simulink library "PRISMA"  (R2025b)
settings: Solver=VariableStepAuto  StartTime=0.0  StopTime=10.0  RelTol=1e-3
libraries: $bdroot x116, etargetslib x30, simulink x9
(part 2 of 3)

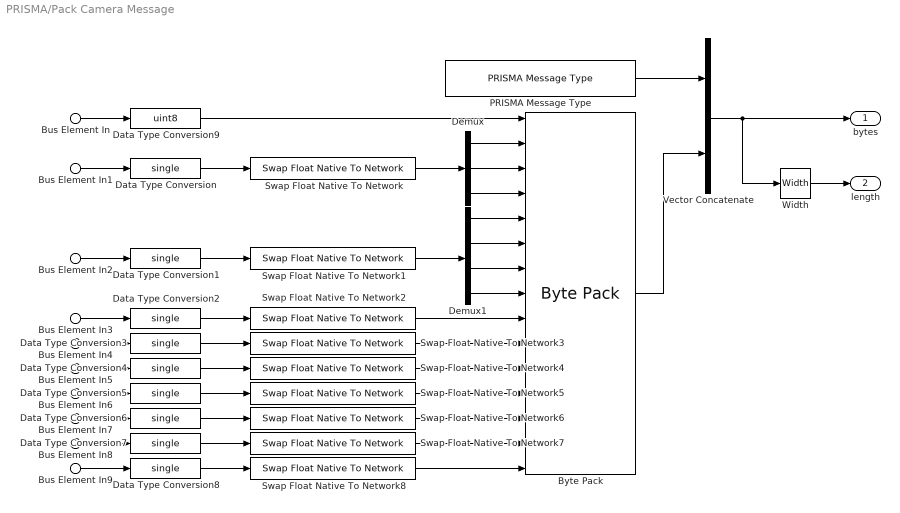
== system PRISMA/Pack Camera Message ==
  Bus Element In : Inport  PortName=camera  Element=mode
  Bus Element In1 : Inport  PortName=camera  Element=position
  Bus Element In2 : Inport  PortName=camera  Element=quaternion
  Bus Element In3 : Inport  PortName=camera  Element=clipNear
  Bus Element In4 : Inport  PortName=camera  Element=clipFar
  Bus Element In5 : Inport  PortName=camera  Element=orthographicLeft
  Bus Element In6 : Inport  PortName=camera  Element=orthographicRight
  Bus Element In7 : Inport  PortName=camera  Element=orthographicBottom
  Bus Element In8 : Inport  PortName=camera  Element=orthographicTop
  Bus Element In9 : Inport  PortName=camera  Element=perspectiveFieldOfView
  Byte Pack : etargetslib/Byte Pack  datatypes={'uint8','single','single','single','single','single','single','single','single','single','single','single','single','single','single'}  byteAlign=1
  Data Type Conversion{,1..8} (9 alike) : DataTypeConversion  OutDataTypeStr=single  SaturateOnIntegerOverflow=off  RndMeth=Floor
  Data Type Conversion9 : DataTypeConversion  OutDataTypeStr=uint8  SaturateOnIntegerOverflow=off  RndMeth=Floor
  Demux : Demux  Outputs=3
  Demux1 : Demux
  PRISMA Message Type : $bdroot/details/PRISMA Message Type  messageType=Camera
  Swap Float Native To Network{,1..8} (9 alike) : $bdroot/details/Swap Float Native To Network
  Vector Concatenate : Concatenate
  Width : Width  DataType=int32
  bytes : Outport  OutDataTypeStr=uint8
  length : Outport  Port=2  OutDataTypeStr=int32  PortDimensions=1
  wires:
  Bus Element In9/1 -> Data Type Conversion8/1
  Bus Element In8/1 -> Data Type Conversion7/1
  Bus Element In7/1 -> Data Type Conversion6/1
  Bus Element In6/1 -> Data Type Conversion5/1
  Bus Element In5/1 -> Data Type Conversion4/1
  Bus Element In4/1 -> Data Type Conversion3/1
  Bus Element In3/1 -> Data Type Conversion2/1
  Data Type Conversion6/1 -> Swap Float Native To Network6/1
  Data Type Conversion8/1 -> Swap Float Native To Network8/1
  Data Type Conversion7/1 -> Swap Float Native To Network7/1
  Data Type Conversion4/1 -> Swap Float Native To Network4/1
  Data Type Conversion5/1 -> Swap Float Native To Network5/1
  Data Type Conversion3/1 -> Swap Float Native To Network3/1
  Data Type Conversion2/1 -> Swap Float Native To Network2/1
  Bus Element In/1 -> Data Type Conversion9/1
  Bus Element In2/1 -> Data Type Conversion1/1
  Data Type Conversion1/1 -> Swap Float Native To Network1/1
  Demux1/4 -> Byte Pack/8
  Demux1/3 -> Byte Pack/7
  Demux1/2 -> Byte Pack/6
  Demux1/1 -> Byte Pack/5
  Bus Element In1/1 -> Data Type Conversion/1
  Demux/3 -> Byte Pack/4
  Demux/2 -> Byte Pack/3
  Demux/1 -> Byte Pack/2
  Data Type Conversion/1 -> Swap Float Native To Network/1
  PRISMA Message Type/1 -> Vector Concatenate/1
  Byte Pack/1 -> Vector Concatenate/2
  Vector Concatenate/1 -> Width/1, bytes/1
  Width/1 -> length/1
  Data Type Conversion9/1 -> Byte Pack/1
  Swap Float Native To Network/1 -> Demux/1
  Swap Float Native To Network1/1 -> Demux1/1
  Swap Float Native To Network2/1 -> Byte Pack/9
  Swap Float Native To Network3/1 -> Byte Pack/10
  Swap Float Native To Network4/1 -> Byte Pack/11
  Swap Float Native To Network5/1 -> Byte Pack/12
  Swap Float Native To Network6/1 -> Byte Pack/13
  Swap Float Native To Network7/1 -> Byte Pack/14
  Swap Float Native To Network8/1 -> Byte Pack/15

== system PRISMA/Pack Clear Message ==
  PRISMA Message Type : $bdroot/details/PRISMA Message Type  messageType=Clear
  Width : Width  DataType=int32
  bytes : Outport  OutDataTypeStr=uint8
  length : Outport  Port=2  OutDataTypeStr=int32  PortDimensions=1
  wires:
  Width/1 -> length/1
  PRISMA Message Type/1 -> bytes/1, Width/1

== system PRISMA/Pack Directional Light Message ==
  Bus Element In : Inport  PortName=directionalLight  Element=shouldBeDeleted
  Bus Element In1 : Inport  PortName=directionalLight  Element=directionalLightID
  Bus Element In2 : Inport  PortName=directionalLight  Element=visible
  Bus Element In3 : Inport  PortName=directionalLight  Element=color
  Bus Element In4 : Inport  PortName=directionalLight  Element=direction
  Byte Pack : etargetslib/Byte Pack  datatypes={'uint32','uint8','single','single','single','single','single','single'}  byteAlign=1
  Constant : Constant  Value=false  OutDataTypeStr=boolean
  Data Type Conversion : DataTypeConversion  OutDataTypeStr=single  SaturateOnIntegerOverflow=off  RndMeth=Floor
  Data Type Conversion1 : DataTypeConversion  OutDataTypeStr=uint32  SaturateOnIntegerOverflow=off  RndMeth=Floor
  Data Type Conversion2 : DataTypeConversion  OutDataTypeStr=single  SaturateOnIntegerOverflow=off  RndMeth=Floor
  Data Type Conversion3 : DataTypeConversion  OutDataTypeStr=boolean  SaturateOnIntegerOverflow=off  RndMeth=Floor
  Data Type Conversion4 : DataTypeConversion  OutDataTypeStr=boolean  SaturateOnIntegerOverflow=off  RndMeth=Floor
  Demux : Demux  Outputs=3
  Demux1 : Demux  Outputs=3
  Mux : Mux  Inputs=8
  PRISMA Bitfield To Byte : $bdroot/details/PRISMA Bitfield To Byte
  PRISMA Message Type : $bdroot/details/PRISMA Message Type  messageType=Directional Light
  Swap Float Native To Network : $bdroot/details/Swap Float Native To Network
  Swap Float Native To Network1 : $bdroot/details/Swap Float Native To Network
  Swap Uint32 Native To Network : $bdroot/details/Swap Uint32 Native To Network
  Vector Concatenate : Concatenate
  Width : Width  DataType=int32
  bytes : Outport  OutDataTypeStr=uint8
  length : Outport  Port=2  OutDataTypeStr=int32  PortDimensions=1
  wires:
  Bus Element In4/1 -> Data Type Conversion2/1
  Bus Element In3/1 -> Data Type Conversion/1
  Demux1/1 -> Byte Pack/6
  Demux1/2 -> Byte Pack/7
  Demux1/3 -> Byte Pack/8
  Demux/1 -> Byte Pack/3
  Demux/2 -> Byte Pack/4
  Demux/3 -> Byte Pack/5
  Data Type Conversion2/1 -> Swap Float Native To Network1/1
  Bus Element In2/1 -> Data Type Conversion4/1
  Bus Element In/1 -> Data Type Conversion3/1
  PRISMA Bitfield To Byte/1 -> Byte Pack/2
  Constant/1 -> Mux/8, Mux/3, Mux/4, Mux/5, Mux/6, Mux/7
  Mux/1 -> PRISMA Bitfield To Byte/1
  Bus Element In1/1 -> Data Type Conversion1/1
  Data Type Conversion1/1 -> Swap Uint32 Native To Network/1
  Data Type Conversion/1 -> Swap Float Native To Network/1
  PRISMA Message Type/1 -> Vector Concatenate/1
  Byte Pack/1 -> Vector Concatenate/2
  Vector Concatenate/1 -> Width/1, bytes/1
  Width/1 -> length/1
  Data Type Conversion3/1 -> Mux/1
  Data Type Conversion4/1 -> Mux/2
  Swap Uint32 Native To Network/1 -> Byte Pack/1
  Swap Float Native To Network/1 -> Demux/1
  Swap Float Native To Network1/1 -> Demux1/1

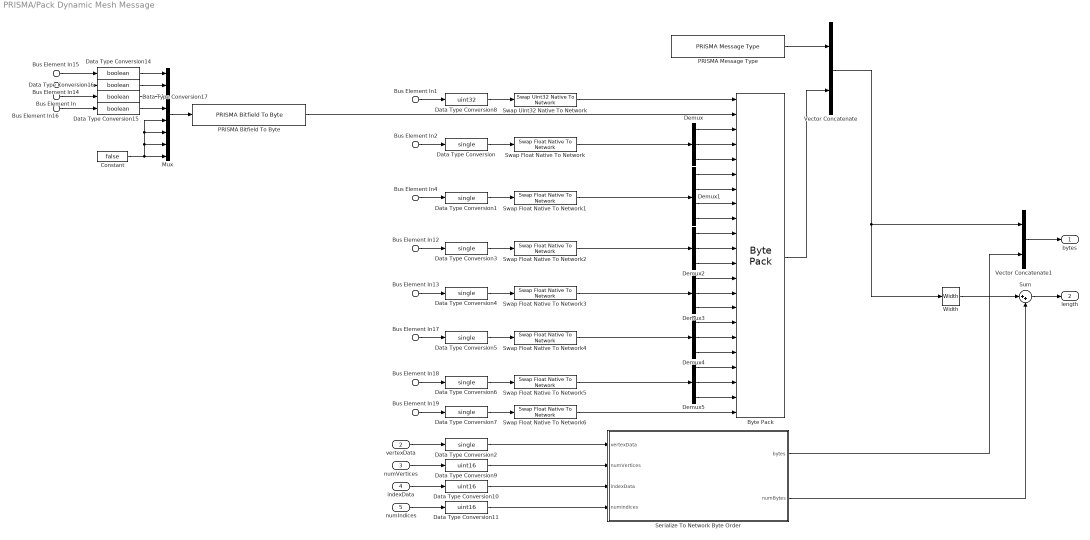
== system PRISMA/Pack Dynamic Mesh Message ==
  Bus Element In14 : Inport  PortName=dynamicMesh  Element=updateMesh
  Bus Element In : Inport  PortName=dynamicMesh  Element=visible
  Bus Element In15 : Inport  PortName=dynamicMesh  Element=shouldBeDeleted
  Bus Element In16 : Inport  PortName=dynamicMesh  Element=castShadow
  Bus Element In1 : Inport  PortName=dynamicMesh  Element=meshID
  Bus Element In2 : Inport  PortName=dynamicMesh  Element=position
  Bus Element In4 : Inport  PortName=dynamicMesh  Element=quaternion
  Bus Element In12 : Inport  PortName=dynamicMesh  Element=scale
  Bus Element In13 : Inport  PortName=dynamicMesh  Element=diffuseColorMultiplier
  Bus Element In17 : Inport  PortName=dynamicMesh  Element=specularColorMultiplier
  Bus Element In18 : Inport  PortName=dynamicMesh  Element=emissionColorMultiplier
  Bus Element In19 : Inport  PortName=dynamicMesh  Element=shininessMultiplier
  vertexData : Inport  Port=2  PortDimensions=[6,2000]
  numVertices : Inport  Port=3  PortDimensions=1
  indexData : Inport  Port=4  PortDimensions=10000
  numIndices : Inport  Port=5  PortDimensions=1
  Byte Pack : etargetslib/Byte Pack  datatypes={'uint32','uint8','single','single','single','single','single','single','single','single','single','single','single','single','single','single','single','single','single','single','single','single'}  byteAlign=1
  Constant : Constant  Value=false  OutDataTypeStr=boolean
  Data Type Conversion{,1..7} (8 alike) : DataTypeConversion  OutDataTypeStr=single  SaturateOnIntegerOverflow=off  RndMeth=Floor
  Data Type Conversion10 : DataTypeConversion  OutDataTypeStr=uint16  SaturateOnIntegerOverflow=off  RndMeth=Floor
  Data Type Conversion11 : DataTypeConversion  OutDataTypeStr=uint16  SaturateOnIntegerOverflow=off  RndMeth=Floor
  Data Type Conversion{14..17} (4 alike) : DataTypeConversion  OutDataTypeStr=boolean  SaturateOnIntegerOverflow=off  RndMeth=Floor
  Data Type Conversion8 : DataTypeConversion  OutDataTypeStr=uint32  SaturateOnIntegerOverflow=off  RndMeth=Floor
  Data Type Conversion9 : DataTypeConversion  OutDataTypeStr=uint16  SaturateOnIntegerOverflow=off  RndMeth=Floor
  Demux{,2..5} (5 alike) : Demux  Outputs=3
  Demux1 : Demux
  Mux : Mux  Inputs=8
  PRISMA Bitfield To Byte : $bdroot/details/PRISMA Bitfield To Byte
  PRISMA Message Type : $bdroot/details/PRISMA Message Type  messageType=Dynamic Mesh
  Serialize To Network Byte Order : MATLAB Function  TreatAsAtomicUnit=on
  Sum : Sum  Inputs=|++
  Swap Float Native To Network{,1..6} (7 alike) : $bdroot/details/Swap Float Native To Network
  Swap Uint32 Native To Network : $bdroot/details/Swap Uint32 Native To Network
  Vector Concatenate : Concatenate
  Vector Concatenate1 : Concatenate
  Width : Width  DataType=int32
  bytes : Outport  OutDataTypeStr=uint8
  length : Outport  Port=2  OutDataTypeStr=int32  PortDimensions=1
  wires:
  Bus Element In14/1 -> Data Type Conversion16/1
  Constant/1 -> Mux/7, Mux/6, Mux/5, Mux/8
  Mux/1 -> PRISMA Bitfield To Byte/1
  Vector Concatenate/1 -> Vector Concatenate1/1, Width/1
  Vector Concatenate1/1 -> bytes/1
  Serialize To Network Byte Order/2(numBytes) -> Sum/2
  Serialize To Network Byte Order/1(bytes) -> Vector Concatenate1/2
  Byte Pack/1 -> Vector Concatenate/2
  Sum/1 -> length/1
  Width/1 -> Sum/1
  Bus Element In/1 -> Data Type Conversion17/1
  PRISMA Message Type/1 -> Vector Concatenate/1
  Data Type Conversion16/1 -> Mux/2
  Data Type Conversion17/1 -> Mux/3
  Data Type Conversion14/1 -> Mux/1
  Bus Element In15/1 -> Data Type Conversion14/1
  Bus Element In16/1 -> Data Type Conversion15/1
  Data Type Conversion15/1 -> Mux/4
  Bus Element In13/1 -> Data Type Conversion4/1
  Bus Element In17/1 -> Data Type Conversion5/1
  Bus Element In19/1 -> Data Type Conversion7/1
  Data Type Conversion7/1 -> Swap Float Native To Network6/1
  Demux1/4 -> Byte Pack/9
  Demux1/1 -> Byte Pack/6
  Demux3/3 -> Byte Pack/15
  Demux1/3 -> Byte Pack/8
  Demux/2 -> Byte Pack/4
  Demux/3 -> Byte Pack/5
  Demux/1 -> Byte Pack/3
  Data Type Conversion6/1 -> Swap Float Native To Network5/1
  Demux3/2 -> Byte Pack/14
  Demux2/3 -> Byte Pack/12
  Demux2/2 -> Byte Pack/11
  Data Type Conversion8/1 -> Swap Uint32 Native To Network/1
  Demux4/2 -> Byte Pack/17
  Data Type Conversion5/1 -> Swap Float Native To Network4/1
  Bus Element In2/1 -> Data Type Conversion/1
  Data Type Conversion3/1 -> Swap Float Native To Network2/1
  Demux5/3 -> Byte Pack/21
  Demux5/2 -> Byte Pack/20
  Bus Element In1/1 -> Data Type Conversion8/1
  Demux2/1 -> Byte Pack/10
  Demux3/1 -> Byte Pack/13
  Demux5/1 -> Byte Pack/19
  PRISMA Bitfield To Byte/1 -> Byte Pack/2
  Data Type Conversion/1 -> Swap Float Native To Network/1
  Demux1/2 -> Byte Pack/7
  Bus Element In18/1 -> Data Type Conversion6/1
  Data Type Conversion4/1 -> Swap Float Native To Network3/1
  Demux4/3 -> Byte Pack/18
  Data Type Conversion1/1 -> Swap Float Native To Network1/1
  Bus Element In4/1 -> Data Type Conversion1/1
  Demux4/1 -> Byte Pack/16
  Bus Element In12/1 -> Data Type Conversion3/1
  vertexData/1 -> Data Type Conversion2/1
  numVertices/1 -> Data Type Conversion9/1
  indexData/1 -> Data Type Conversion10/1
  numIndices/1 -> Data Type Conversion11/1
  Swap Uint32 Native To Network/1 -> Byte Pack/1
  Swap Float Native To Network/1 -> Demux/1
  Swap Float Native To Network1/1 -> Demux1/1
  Swap Float Native To Network2/1 -> Demux2/1
  Swap Float Native To Network3/1 -> Demux3/1
  Swap Float Native To Network4/1 -> Demux4/1
  Swap Float Native To Network5/1 -> Demux5/1
  Swap Float Native To Network6/1 -> Byte Pack/22
  Data Type Conversion2/1 -> Serialize To Network Byte Order/1(vertexData)
  Data Type Conversion9/1 -> Serialize To Network Byte Order/2(numVertices)
  Data Type Conversion10/1 -> Serialize To Network Byte Order/3(indexData)
  Data Type Conversion11/1 -> Serialize To Network Byte Order/4(numIndices)

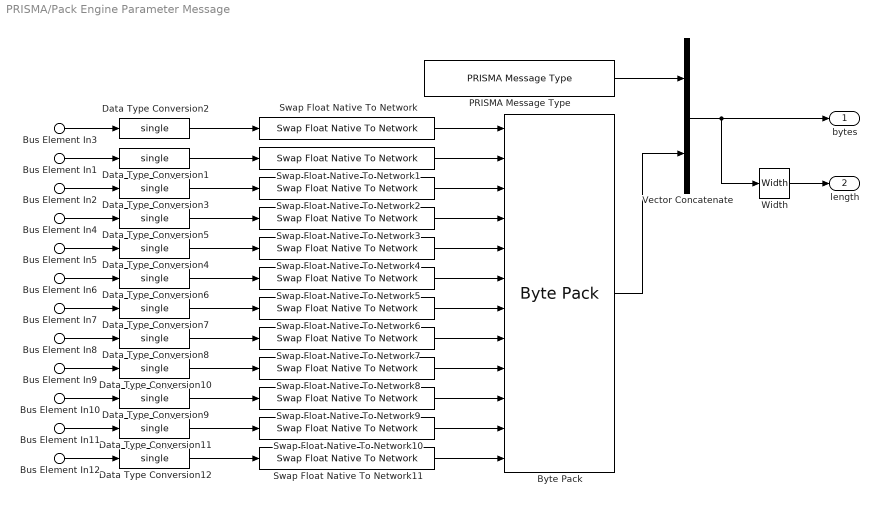
== system PRISMA/Pack Engine Parameter Message ==
  Bus Element In3 : Inport  PortName=engineParameter  Element=ambientOcclusionRadius
  Bus Element In1 : Inport  PortName=engineParameter  Element=ambientOcclusionBias
  Bus Element In2 : Inport  PortName=engineParameter  Element=ambientOcclusionEnhance
  Bus Element In4 : Inport  PortName=engineParameter  Element=removeShadowOnWater
  Bus Element In5 : Inport  PortName=engineParameter  Element=bloomBrightnessThreshold
  Bus Element In6 : Inport  PortName=engineParameter  Element=bloomStrength
  Bus Element In7 : Inport  PortName=engineParameter  Element=gamma
  Bus Element In8 : Inport  PortName=engineParameter  Element=ditheringNoiseGranularity
  Bus Element In9 : Inport  PortName=engineParameter  Element=shadowBiasMin
  Bus Element In10 : Inport  PortName=engineParameter  Element=shadowBiasMax
  Bus Element In11 : Inport  PortName=engineParameter  Element=exposure
  Bus Element In12 : Inport  PortName=engineParameter  Element=toneMappingStrength
  Byte Pack : etargetslib/Byte Pack  datatypes={'single','single','single','single','single','single','single','single','single','single','single','single'}  byteAlign=1
  Data Type Conversion{1..12} (12 alike) : DataTypeConversion  OutDataTypeStr=single  SaturateOnIntegerOverflow=off  RndMeth=Floor
  PRISMA Message Type : $bdroot/details/PRISMA Message Type  messageType=Engine Parameter
  Swap Float Native To Network{,1..11} (12 alike) : $bdroot/details/Swap Float Native To Network
  Vector Concatenate : Concatenate
  Width : Width  DataType=int32
  bytes : Outport  OutDataTypeStr=uint8
  length : Outport  Port=2  OutDataTypeStr=int32  PortDimensions=1
  wires:
  Bus Element In12/1 -> Data Type Conversion12/1
  Bus Element In11/1 -> Data Type Conversion11/1
  Bus Element In10/1 -> Data Type Conversion9/1
  Bus Element In9/1 -> Data Type Conversion10/1
  Bus Element In8/1 -> Data Type Conversion8/1
  Bus Element In7/1 -> Data Type Conversion7/1
  Bus Element In6/1 -> Data Type Conversion6/1
  Bus Element In5/1 -> Data Type Conversion4/1
  Bus Element In4/1 -> Data Type Conversion5/1
  Bus Element In2/1 -> Data Type Conversion3/1
  Bus Element In1/1 -> Data Type Conversion1/1
  Width/1 -> length/1
  Vector Concatenate/1 -> bytes/1, Width/1
  Byte Pack/1 -> Vector Concatenate/2
  PRISMA Message Type/1 -> Vector Concatenate/1
  Bus Element In3/1 -> Data Type Conversion2/1
  Data Type Conversion2/1 -> Swap Float Native To Network/1
  Data Type Conversion1/1 -> Swap Float Native To Network1/1
  Data Type Conversion3/1 -> Swap Float Native To Network2/1
  Data Type Conversion5/1 -> Swap Float Native To Network3/1
  Data Type Conversion4/1 -> Swap Float Native To Network4/1
  Data Type Conversion6/1 -> Swap Float Native To Network5/1
  Data Type Conversion7/1 -> Swap Float Native To Network6/1
  Data Type Conversion8/1 -> Swap Float Native To Network7/1
  Data Type Conversion10/1 -> Swap Float Native To Network8/1
  Data Type Conversion9/1 -> Swap Float Native To Network9/1
  Data Type Conversion11/1 -> Swap Float Native To Network10/1
  Data Type Conversion12/1 -> Swap Float Native To Network11/1
  Swap Float Native To Network/1 -> Byte Pack/1
  Swap Float Native To Network1/1 -> Byte Pack/2
  Swap Float Native To Network2/1 -> Byte Pack/3
  Swap Float Native To Network3/1 -> Byte Pack/4
  Swap Float Native To Network4/1 -> Byte Pack/5
  Swap Float Native To Network5/1 -> Byte Pack/6
  Swap Float Native To Network6/1 -> Byte Pack/7
  Swap Float Native To Network7/1 -> Byte Pack/8
  Swap Float Native To Network8/1 -> Byte Pack/9
  Swap Float Native To Network9/1 -> Byte Pack/10
  Swap Float Native To Network10/1 -> Byte Pack/11
  Swap Float Native To Network11/1 -> Byte Pack/12

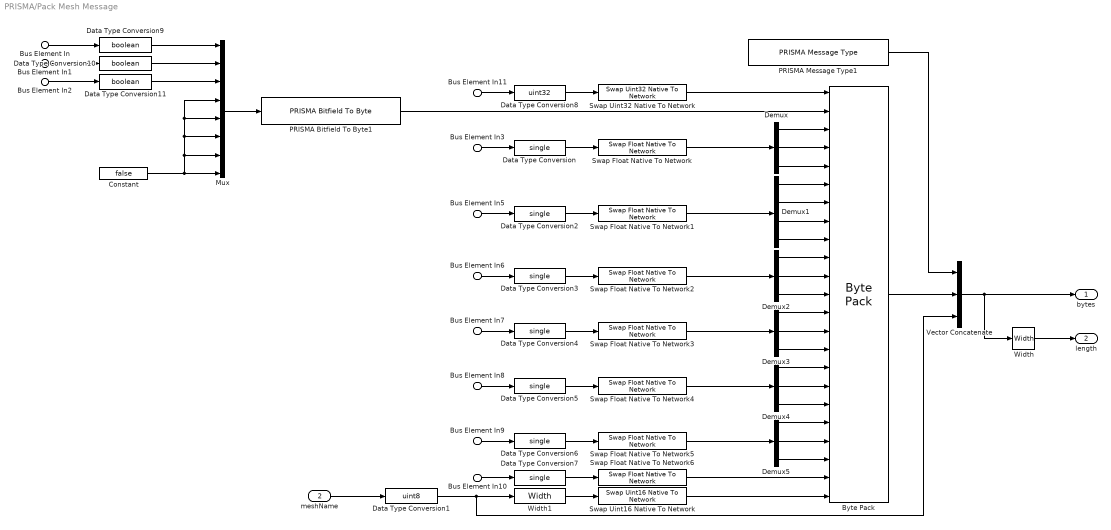
== system PRISMA/Pack Mesh Message ==
  Bus Element In : Inport  PortName=mesh  Element=shouldBeDeleted
  Bus Element In1 : Inport  PortName=mesh  Element=visible
  Bus Element In2 : Inport  PortName=mesh  Element=castShadow
  Bus Element In3 : Inport  PortName=mesh  Element=position
  Bus Element In5 : Inport  PortName=mesh  Element=quaternion
  Bus Element In6 : Inport  PortName=mesh  Element=scale
  Bus Element In7 : Inport  PortName=mesh  Element=diffuseColorMultiplier
  Bus Element In8 : Inport  PortName=mesh  Element=specularColorMultiplier
  Bus Element In9 : Inport  PortName=mesh  Element=emissionColorMultiplier
  Bus Element In10 : Inport  PortName=mesh  Element=shininessMultiplier
  Bus Element In11 : Inport  PortName=mesh  Element=meshID
  meshName : Inport  Port=2  OutDataTypeStr=uint8
  Byte Pack : etargetslib/Byte Pack  datatypes={'uint32','uint8','single','single','single','single','single','single','single','single','single','single','single','single','single','single','single','single','single','single','single','single','uint16'}  byteAlign=1
  Constant : Constant  Value=false  OutDataTypeStr=boolean
  Data Type Conversion{,2..7} (7 alike) : DataTypeConversion  OutDataTypeStr=single  SaturateOnIntegerOverflow=off  RndMeth=Floor
  Data Type Conversion1 : DataTypeConversion  OutDataTypeStr=uint8  SaturateOnIntegerOverflow=off  RndMeth=Floor
  Data Type Conversion10 : DataTypeConversion  OutDataTypeStr=boolean  SaturateOnIntegerOverflow=off  RndMeth=Floor
  Data Type Conversion11 : DataTypeConversion  OutDataTypeStr=boolean  SaturateOnIntegerOverflow=off  RndMeth=Floor
  Data Type Conversion8 : DataTypeConversion  OutDataTypeStr=uint32  SaturateOnIntegerOverflow=off  RndMeth=Floor
  Data Type Conversion9 : DataTypeConversion  OutDataTypeStr=boolean  SaturateOnIntegerOverflow=off  RndMeth=Floor
  Demux{,2..5} (5 alike) : Demux  Outputs=3
  Demux1 : Demux
  Mux : Mux  Inputs=8
  PRISMA Bitfield To Byte1 : $bdroot/details/PRISMA Bitfield To Byte
  PRISMA Message Type1 : $bdroot/details/PRISMA Message Type  messageType=Mesh
  Swap Float Native To Network{,1..6} (7 alike) : $bdroot/details/Swap Float Native To Network
  Swap Uint16 Native To Network : $bdroot/details/Swap Uint16 Native To Network
  Swap Uint32 Native To Network : $bdroot/details/Swap Uint32 Native To Network
  Vector Concatenate : Concatenate  NumInputs=3
  Width : Width  DataType=int32
  Width1 : Width  DataType=uint16
  bytes : Outport  OutDataTypeStr=uint8
  length : Outport  Port=2  OutDataTypeStr=int32  PortDimensions=1
  wires:
  Data Type Conversion8/1 -> Swap Uint32 Native To Network/1
  Bus Element In10/1 -> Data Type Conversion7/1
  Bus Element In9/1 -> Data Type Conversion6/1
  Bus Element In8/1 -> Data Type Conversion5/1
  Bus Element In7/1 -> Data Type Conversion4/1
  Bus Element In6/1 -> Data Type Conversion3/1
  Bus Element In5/1 -> Data Type Conversion2/1
  Bus Element In3/1 -> Data Type Conversion/1
  Bus Element In2/1 -> Data Type Conversion11/1
  Bus Element In/1 -> Data Type Conversion9/1
  Width/1 -> length/1
  Vector Concatenate/1 -> bytes/1, Width/1
  Width1/1 -> Swap Uint16 Native To Network/1
  Data Type Conversion7/1 -> Swap Float Native To Network6/1
  Data Type Conversion6/1 -> Swap Float Native To Network5/1
  Data Type Conversion5/1 -> Swap Float Native To Network4/1
  Data Type Conversion4/1 -> Swap Float Native To Network3/1
  Data Type Conversion3/1 -> Swap Float Native To Network2/1
  Data Type Conversion2/1 -> Swap Float Native To Network1/1
  Data Type Conversion/1 -> Swap Float Native To Network/1
  Mux/1 -> PRISMA Bitfield To Byte1/1
  Constant/1 -> Mux/4, Mux/5, Mux/6, Mux/7, Mux/8
  Bus Element In1/1 -> Data Type Conversion10/1
  PRISMA Bitfield To Byte1/1 -> Byte Pack/2
  meshName/1 -> Data Type Conversion1/1
  Demux5/3 -> Byte Pack/21
  Demux5/2 -> Byte Pack/20
  Demux5/1 -> Byte Pack/19
  Demux4/1 -> Byte Pack/16
  Demux4/2 -> Byte Pack/17
  Demux4/3 -> Byte Pack/18
  Demux3/3 -> Byte Pack/15
  Demux3/2 -> Byte Pack/14
  Demux3/1 -> Byte Pack/13
  Demux2/1 -> Byte Pack/10
  Demux2/2 -> Byte Pack/11
  Demux2/3 -> Byte Pack/12
  Demux/3 -> Byte Pack/5
  Demux/2 -> Byte Pack/4
  Demux/1 -> Byte Pack/3
  Byte Pack/1 -> Vector Concatenate/2
  PRISMA Message Type1/1 -> Vector Concatenate/1
  Bus Element In11/1 -> Data Type Conversion8/1
  Demux1/4 -> Byte Pack/9
  Demux1/3 -> Byte Pack/8
  Demux1/2 -> Byte Pack/7
  Demux1/1 -> Byte Pack/6
  Data Type Conversion1/1 -> Vector Concatenate/3, Width1/1
  Data Type Conversion9/1 -> Mux/1
  Data Type Conversion10/1 -> Mux/2
  Data Type Conversion11/1 -> Mux/3
  Swap Uint32 Native To Network/1 -> Byte Pack/1
  Swap Float Native To Network/1 -> Demux/1
  Swap Float Native To Network1/1 -> Demux1/1
  Swap Float Native To Network2/1 -> Demux2/1
  Swap Float Native To Network3/1 -> Demux3/1
  Swap Float Native To Network4/1 -> Demux4/1
  Swap Float Native To Network5/1 -> Demux5/1
  Swap Float Native To Network6/1 -> Byte Pack/22
  Swap Uint16 Native To Network/1 -> Byte Pack/23

== system PRISMA/Pack Point Light Message ==
  Bus Element In : Inport  PortName=pointLight  Element=shouldBeDeleted
  Bus Element In1 : Inport  PortName=pointLight  Element=pointLightID
  Bus Element In2 : Inport  PortName=pointLight  Element=visible
  Bus Element In3 : Inport  PortName=pointLight  Element=color
  Bus Element In4 : Inport  PortName=pointLight  Element=position
  Bus Element In5 : Inport  PortName=pointLight  Element=quadraticFalloff
  Bus Element In6 : Inport  PortName=pointLight  Element=invRadiusPow4
  Byte Pack : etargetslib/Byte Pack  datatypes={'uint32','uint8','single','single','single','single','single','single','single','single'}  byteAlign=1
  Constant : Constant  Value=false  OutDataTypeStr=boolean
  Data Type Conversion{,2..4} (4 alike) : DataTypeConversion  OutDataTypeStr=single  SaturateOnIntegerOverflow=off  RndMeth=Floor
  Data Type Conversion1 : DataTypeConversion  OutDataTypeStr=uint32  SaturateOnIntegerOverflow=off  RndMeth=Floor
  Data Type Conversion5 : DataTypeConversion  OutDataTypeStr=boolean  SaturateOnIntegerOverflow=off  RndMeth=Floor
  Data Type Conversion6 : DataTypeConversion  OutDataTypeStr=boolean  SaturateOnIntegerOverflow=off  RndMeth=Floor
  Demux1 : Demux  Outputs=3
  Demux2 : Demux  Outputs=3
  Mux : Mux  Inputs=8
  PRISMA Bitfield To Byte : $bdroot/details/PRISMA Bitfield To Byte
  PRISMA Message Type : $bdroot/details/PRISMA Message Type  messageType=Point Light
  Swap Float Native To Network{,1..3} (4 alike) : $bdroot/details/Swap Float Native To Network
  Swap Uint32 Native To Network : $bdroot/details/Swap Uint32 Native To Network
  Vector Concatenate : Concatenate
  Width : Width  DataType=int32
  bytes : Outport  OutDataTypeStr=uint8
  length : Outport  Port=2  OutDataTypeStr=int32  PortDimensions=1
  wires:
  Data Type Conversion/1 -> Swap Float Native To Network/1
  Demux2/3 -> Byte Pack/5
  Demux2/2 -> Byte Pack/4
  Demux2/1 -> Byte Pack/3
  Data Type Conversion4/1 -> Swap Float Native To Network3/1
  Bus Element In6/1 -> Data Type Conversion4/1
  Bus Element In5/1 -> Data Type Conversion3/1
  Data Type Conversion3/1 -> Swap Float Native To Network2/1
  Width/1 -> length/1
  Vector Concatenate/1 -> bytes/1, Width/1
  Byte Pack/1 -> Vector Concatenate/2
  PRISMA Message Type/1 -> Vector Concatenate/1
  Data Type Conversion1/1 -> Swap Uint32 Native To Network/1
  Bus Element In1/1 -> Data Type Conversion1/1
  Mux/1 -> PRISMA Bitfield To Byte/1
  Constant/1 -> Mux/7, Mux/6, Mux/5, Mux/4, Mux/3, Mux/8
  PRISMA Bitfield To Byte/1 -> Byte Pack/2
  Bus Element In/1 -> Data Type Conversion5/1
  Bus Element In2/1 -> Data Type Conversion6/1
  Data Type Conversion2/1 -> Swap Float Native To Network1/1
  Demux1/3 -> Byte Pack/8
  Demux1/2 -> Byte Pack/7
  Demux1/1 -> Byte Pack/6
  Bus Element In3/1 -> Data Type Conversion/1
  Bus Element In4/1 -> Data Type Conversion2/1
  Data Type Conversion5/1 -> Mux/1
  Data Type Conversion6/1 -> Mux/2
  Swap Uint32 Native To Network/1 -> Byte Pack/1
  Swap Float Native To Network/1 -> Demux2/1
  Swap Float Native To Network1/1 -> Demux1/1
  Swap Float Native To Network2/1 -> Byte Pack/9
  Swap Float Native To Network3/1 -> Byte Pack/10

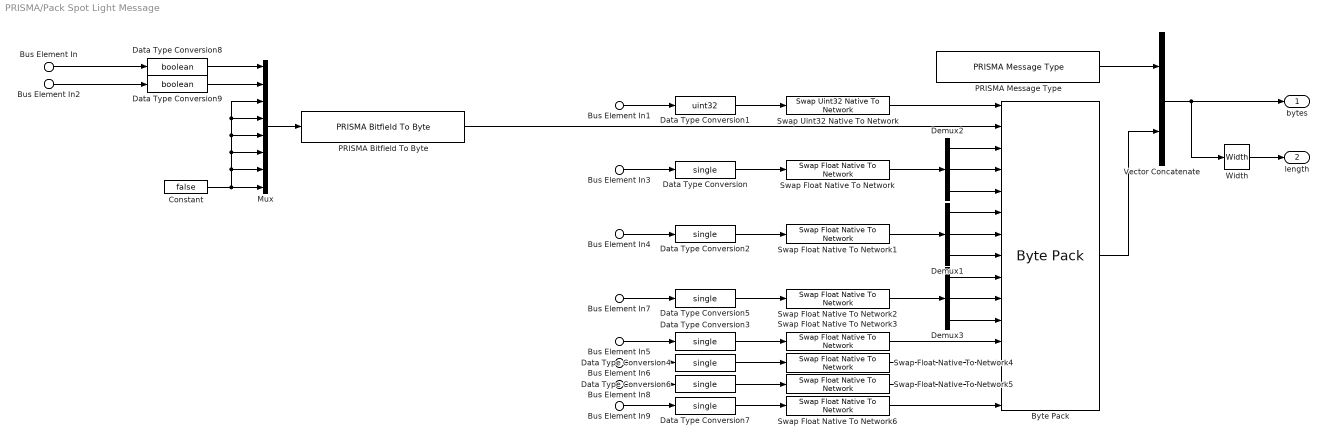
== system PRISMA/Pack Spot Light Message ==
  Bus Element In : Inport  PortName=spotLight  Element=shouldBeDeleted
  Bus Element In1 : Inport  PortName=spotLight  Element=spotLightID
  Bus Element In2 : Inport  PortName=spotLight  Element=visible
  Bus Element In3 : Inport  PortName=spotLight  Element=color
  Bus Element In4 : Inport  PortName=spotLight  Element=position
  Bus Element In5 : Inport  PortName=spotLight  Element=quadraticFalloff
  Bus Element In6 : Inport  PortName=spotLight  Element=invRadiusPow4
  Bus Element In7 : Inport  PortName=spotLight  Element=direction
  Bus Element In8 : Inport  PortName=spotLight  Element=cosInnerCutOffAngle
  Bus Element In9 : Inport  PortName=spotLight  Element=cosOuterCutOffAngle
  Byte Pack : etargetslib/Byte Pack  datatypes={'uint32','uint8','single','single','single','single','single','single','single','single','single','single','single','single','single'}  byteAlign=1
  Constant : Constant  Value=false  OutDataTypeStr=boolean
  Data Type Conversion{,2..7} (7 alike) : DataTypeConversion  OutDataTypeStr=single  SaturateOnIntegerOverflow=off  RndMeth=Floor
  Data Type Conversion1 : DataTypeConversion  OutDataTypeStr=uint32  SaturateOnIntegerOverflow=off  RndMeth=Floor
  Data Type Conversion8 : DataTypeConversion  OutDataTypeStr=boolean  SaturateOnIntegerOverflow=off  RndMeth=Floor
  Data Type Conversion9 : DataTypeConversion  OutDataTypeStr=boolean  SaturateOnIntegerOverflow=off  RndMeth=Floor
  Demux1 : Demux  Outputs=3
  Demux2 : Demux  Outputs=3
  Demux3 : Demux  Outputs=3
  Mux : Mux  Inputs=8
  PRISMA Bitfield To Byte : $bdroot/details/PRISMA Bitfield To Byte
  PRISMA Message Type : $bdroot/details/PRISMA Message Type  messageType=Spot Light
  Swap Float Native To Network{,1..6} (7 alike) : $bdroot/details/Swap Float Native To Network
  Swap Uint32 Native To Network : $bdroot/details/Swap Uint32 Native To Network
  Vector Concatenate : Concatenate
  Width : Width  DataType=int32
  bytes : Outport  OutDataTypeStr=uint8
  length : Outport  Port=2  OutDataTypeStr=int32  PortDimensions=1
  wires:
  Bus Element In9/1 -> Data Type Conversion7/1
  Bus Element In8/1 -> Data Type Conversion6/1
  Data Type Conversion6/1 -> Swap Float Native To Network5/1
  Data Type Conversion7/1 -> Swap Float Native To Network6/1
  Data Type Conversion4/1 -> Swap Float Native To Network4/1
  Data Type Conversion3/1 -> Swap Float Native To Network3/1
  Demux3/3 -> Byte Pack/11
  Demux3/2 -> Byte Pack/10
  Demux3/1 -> Byte Pack/9
  Data Type Conversion5/1 -> Swap Float Native To Network2/1
  Bus Element In7/1 -> Data Type Conversion5/1
  Bus Element In4/1 -> Data Type Conversion2/1
  Bus Element In3/1 -> Data Type Conversion/1
  Demux1/1 -> Byte Pack/6
  Demux1/2 -> Byte Pack/7
  Demux1/3 -> Byte Pack/8
  Data Type Conversion2/1 -> Swap Float Native To Network1/1
  Bus Element In2/1 -> Data Type Conversion9/1
  Bus Element In/1 -> Data Type Conversion8/1
  PRISMA Bitfield To Byte/1 -> Byte Pack/2
  Constant/1 -> Mux/8, Mux/3, Mux/4, Mux/5, Mux/6, Mux/7
  Mux/1 -> PRISMA Bitfield To Byte/1
  Bus Element In1/1 -> Data Type Conversion1/1
  Data Type Conversion1/1 -> Swap Uint32 Native To Network/1
  PRISMA Message Type/1 -> Vector Concatenate/1
  Byte Pack/1 -> Vector Concatenate/2
  Vector Concatenate/1 -> Width/1, bytes/1
  Width/1 -> length/1
  Bus Element In5/1 -> Data Type Conversion3/1
  Bus Element In6/1 -> Data Type Conversion4/1
  Demux2/1 -> Byte Pack/3
  Demux2/2 -> Byte Pack/4
  Demux2/3 -> Byte Pack/5
  Data Type Conversion/1 -> Swap Float Native To Network/1
  Data Type Conversion8/1 -> Mux/1
  Data Type Conversion9/1 -> Mux/2
  Swap Uint32 Native To Network/1 -> Byte Pack/1
  Swap Float Native To Network/1 -> Demux2/1
  Swap Float Native To Network1/1 -> Demux1/1
  Swap Float Native To Network2/1 -> Demux3/1
  Swap Float Native To Network3/1 -> Byte Pack/12
  Swap Float Native To Network4/1 -> Byte Pack/13
  Swap Float Native To Network5/1 -> Byte Pack/14
  Swap Float Native To Network6/1 -> Byte Pack/15

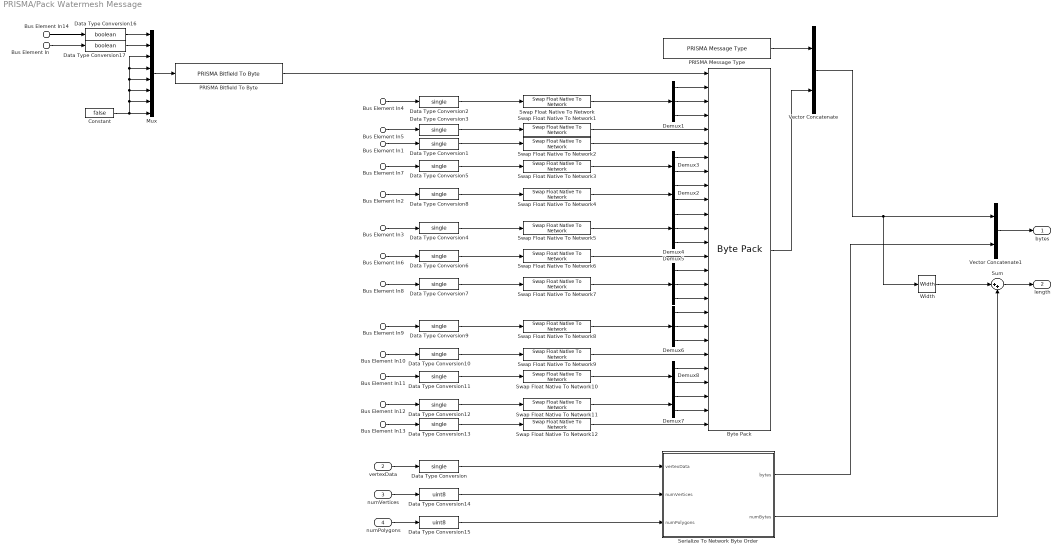
== system PRISMA/Pack Watermesh Message ==
  Bus Element In14 : Inport  PortName=watermesh  Element=updateMesh
  Bus Element In4 : Inport  PortName=watermesh  Element=position
  Bus Element In7 : Inport  PortName=watermesh  Element=textureCoordinateAnimation1
  Bus Element In5 : Inport  PortName=watermesh  Element=textureCoordinateScaling1
  Bus Element In1 : Inport  PortName=watermesh  Element=textureCoordinateScaling2
  Bus Element In2 : Inport  PortName=watermesh  Element=textureCoordinateAnimation2
  Bus Element In3 : Inport  PortName=watermesh  Element=specularColor
  Bus Element In6 : Inport  PortName=watermesh  Element=shininess
  Bus Element In8 : Inport  PortName=watermesh  Element=reflectionColorMultiplier
  Bus Element In9 : Inport  PortName=watermesh  Element=refractionColorMultiplier
  Bus Element In10 : Inport  PortName=watermesh  Element=clippingPlaneOffset
  Bus Element In11 : Inport  PortName=watermesh  Element=strengthDuDvNormal1
  Bus Element In12 : Inport  PortName=watermesh  Element=strengthDuDvNormal2
  Bus Element In13 : Inport  PortName=watermesh  Element=distortionWaterDepthScale
  Bus Element In : Inport  PortName=watermesh  Element=visible
  vertexData : Inport  Port=2  PortDimensions=[2,255,32]
  numVertices : Inport  Port=3  PortDimensions=32
  numPolygons : Inport  Port=4  PortDimensions=1
  Byte Pack : etargetslib/Byte Pack  datatypes={'uint8','single','single','single','single','single','single','single','single','single','single','single','single','single','single','single','single','single','single','single','single','single','single','single','single','single'}  byteAlign=1
  Constant : Constant  Value=false  OutDataTypeStr=boolean
  Data Type Conversion{,1..13} (14 alike) : DataTypeConversion  OutDataTypeStr=single  SaturateOnIntegerOverflow=off  RndMeth=Floor
  Data Type Conversion14 : DataTypeConversion  OutDataTypeStr=uint8  SaturateOnIntegerOverflow=off  RndMeth=Floor
  Data Type Conversion15 : DataTypeConversion  OutDataTypeStr=uint8  SaturateOnIntegerOverflow=off  RndMeth=Floor
  Data Type Conversion16 : DataTypeConversion  OutDataTypeStr=boolean  SaturateOnIntegerOverflow=off  RndMeth=Floor
  Data Type Conversion17 : DataTypeConversion  OutDataTypeStr=boolean  SaturateOnIntegerOverflow=off  RndMeth=Floor
  Demux{1,4..6} (4 alike) : Demux  Outputs=3
  Demux{2..3,7..8} (4 alike) : Demux  Outputs=2
  Mux : Mux  Inputs=8
  PRISMA Bitfield To Byte : $bdroot/details/PRISMA Bitfield To Byte
  PRISMA Message Type : $bdroot/details/PRISMA Message Type  messageType=Watermesh
  Serialize To Network Byte Order : MATLAB Function  TreatAsAtomicUnit=on
  Sum : Sum  Inputs=|++
  Swap Float Native To Network{,1..12} (13 alike) : $bdroot/details/Swap Float Native To Network
  Vector Concatenate : Concatenate
  Vector Concatenate1 : Concatenate
  Width : Width  DataType=int32
  bytes : Outport  OutDataTypeStr=uint8
  length : Outport  Port=2  OutDataTypeStr=int32  PortDimensions=1
  wires:
  Sum/1 -> length/1
  Vector Concatenate1/1 -> bytes/1
  Serialize To Network Byte Order/2(numBytes) -> Sum/2
  Width/1 -> Sum/1
  Serialize To Network Byte Order/1(bytes) -> Vector Concatenate1/2
  numPolygons/1 -> Data Type Conversion15/1
  numVertices/1 -> Data Type Conversion14/1
  vertexData/1 -> Data Type Conversion/1
  Data Type Conversion15/1 -> Serialize To Network Byte Order/3(numPolygons)
  Data Type Conversion14/1 -> Serialize To Network Byte Order/2(numVertices)
  Data Type Conversion13/1 -> Swap Float Native To Network12/1
  Bus Element In13/1 -> Data Type Conversion13/1
  Data Type Conversion11/1 -> Swap Float Native To Network10/1
  Bus Element In11/1 -> Data Type Conversion11/1
  Demux8/1 -> Byte Pack/22
  Demux8/2 -> Byte Pack/23
  Demux7/2 -> Byte Pack/25
  Demux7/1 -> Byte Pack/24
  Bus Element In12/1 -> Data Type Conversion12/1
  Data Type Conversion12/1 -> Swap Float Native To Network11/1
  Data Type Conversion10/1 -> Swap Float Native To Network9/1
  Bus Element In10/1 -> Data Type Conversion10/1
  Demux6/3 -> Byte Pack/20
  Demux6/2 -> Byte Pack/19
  Demux6/1 -> Byte Pack/18
  Data Type Conversion9/1 -> Swap Float Native To Network8/1
  Bus Element In9/1 -> Data Type Conversion9/1
  Bus Element In8/1 -> Data Type Conversion7/1
  Data Type Conversion7/1 -> Swap Float Native To Network7/1
  Demux5/1 -> Byte Pack/15
  Demux5/2 -> Byte Pack/16
  Demux5/3 -> Byte Pack/17
  Bus Element In6/1 -> Data Type Conversion6/1
  Data Type Conversion6/1 -> Swap Float Native To Network6/1
  Bus Element In3/1 -> Data Type Conversion4/1
  Data Type Conversion4/1 -> Swap Float Native To Network5/1
  Demux4/1 -> Byte Pack/11
  Demux4/2 -> Byte Pack/12
  Demux4/3 -> Byte Pack/13
  Data Type Conversion8/1 -> Swap Float Native To Network4/1
  Bus Element In2/1 -> Data Type Conversion8/1
  Demux2/1 -> Byte Pack/9
  Demux2/2 -> Byte Pack/10
  Demux3/2 -> Byte Pack/8
  Demux3/1 -> Byte Pack/7
  Bus Element In1/1 -> Data Type Conversion1/1
  Data Type Conversion1/1 -> Swap Float Native To Network2/1
  Data Type Conversion3/1 -> Swap Float Native To Network1/1
  Demux1/3 -> Byte Pack/4
  Demux1/2 -> Byte Pack/3
  Demux1/1 -> Byte Pack/2
  PRISMA Bitfield To Byte/1 -> Byte Pack/1
  Bus Element In5/1 -> Data Type Conversion3/1
  Vector Concatenate/1 -> Vector Concatenate1/1, Width/1
  Byte Pack/1 -> Vector Concatenate/2
  PRISMA Message Type/1 -> Vector Concatenate/1
  Mux/1 -> PRISMA Bitfield To Byte/1
  Constant/1 -> Mux/7, Mux/6, Mux/5, Mux/4, Mux/3, Mux/8
  Data Type Conversion2/1 -> Swap Float Native To Network/1
  Bus Element In4/1 -> Data Type Conversion2/1
  Bus Element In7/1 -> Data Type Conversion5/1
  Data Type Conversion5/1 -> Swap Float Native To Network3/1
  Data Type Conversion16/1 -> Mux/1
  Data Type Conversion17/1 -> Mux/2
  Bus Element In/1 -> Data Type Conversion17/1
  Bus Element In14/1 -> Data Type Conversion16/1
  Swap Float Native To Network/1 -> Demux1/1
  Swap Float Native To Network1/1 -> Byte Pack/5
  Swap Float Native To Network2/1 -> Byte Pack/6
  Swap Float Native To Network3/1 -> Demux3/1
  Swap Float Native To Network4/1 -> Demux2/1
  Swap Float Native To Network5/1 -> Demux4/1
  Swap Float Native To Network6/1 -> Byte Pack/14
  Swap Float Native To Network7/1 -> Demux5/1
  Swap Float Native To Network8/1 -> Demux6/1
  Swap Float Native To Network9/1 -> Byte Pack/21
  Swap Float Native To Network10/1 -> Demux8/1
  Swap Float Native To Network11/1 -> Demux7/1
  Swap Float Native To Network12/1 -> Byte Pack/26
  Data Type Conversion/1 -> Serialize To Network Byte Order/1(vertexData)

== system PRISMA/Sun Light Color ==
  eyePosition : Inport  OutDataTypeStr=double  Unit=m  PortDimensions=3
  sunLightDirection : Inport  Port=2  OutDataTypeStr=double  PortDimensions=3
  radiusPlanet : Inport  Port=3  OutDataTypeStr=double  Unit=m  PortDimensions=1
  radiusAtmosphere : Inport  Port=4  OutDataTypeStr=double  Unit=m  PortDimensions=1
  scaleHeightRayleigh : Inport  Port=5  OutDataTypeStr=double  Unit=m  PortDimensions=1
  coefficientRayleigh : Inport  Port=6  OutDataTypeStr=double  Unit=1/m  PortDimensions=3
  sunIntensity : Inport  Port=7  OutDataTypeStr=double  PortDimensions=1
  MATLAB Function1 : MATLAB Function  TreatAsAtomicUnit=on
  sunLightColor : Outport  OutDataTypeStr=double  PortDimensions=3
  wires:
  eyePosition/1 -> MATLAB Function1/1(eyePosition)
  MATLAB Function1/1(lightColor) -> sunLightColor/1
  sunLightDirection/1 -> MATLAB Function1/2(sunLightDirection)
  radiusPlanet/1 -> MATLAB Function1/3(radiusPlanet)
  radiusAtmosphere/1 -> MATLAB Function1/4(radiusAtmosphere)
  scaleHeightRayleigh/1 -> MATLAB Function1/5(scaleHeightRayleigh)
  coefficientRayleigh/1 -> MATLAB Function1/6(coefficientRayleigh)
  sunIntensity/1 -> MATLAB Function1/7(sunIntensity)

== system PRISMA/Transformation ==
  Euler ZYX to Quaternion : Subsystem
      mask help: Convert euler angles, given in ZYX convention, to a corresponding unit quaternion. The unit quaternion is given by the components [w;x;y;z], where w denotes the scalar part and [x;y;z] indicates the vector part.
      mask DialogControl DescGroupVar Prompt: EulerZYX to Quaternion
      mask Display:
      | text(0.5, 0.5, '{\bfPRISMA}','horizontalAlignment','center','verticalAlignment','bottom','texmode','on');
      | text(0.5, 0.5, 'Euler (ZYX) to Quaternion','horizontalAlignment','center','verticalAlignment','top');
  Look At to Quaternion : Subsystem
      mask help: Calculate the quaternion based on a given eye position looking to a distant point. The coordinate system is defined to be the NED frame. The quaternion represents a pitch and yaw angle such that a camera located at the eyePosition is looking at the lookAtPosition with a roll angle of zero. The output quaternion is given by [w;x;y;z] where w indicates the scalar component and [x;y;z] represents the vector part.
      mask DialogControl DescGroupVar Prompt: Look At to Quaternion
      mask Display:
      | text(0.5, 0.5, '{\bfPRISMA}','horizontalAlignment','center','verticalAlignment','bottom','texmode','on');
      | text(0.5, 0.5, 'Look At to Quaternion\n(NED)','horizontalAlignment','center','verticalAlignment','top');
  Quaternion to Rotation Matrix : Subsystem
      mask help: Convert a unit quaternion [w;x;y;z] to a corresponding 3-by-3 rotation matrix, where w denotes the scalar part and [x;y;z] indicates the vector part of the unit quaternion.
      mask DialogControl DescGroupVar Prompt: Quaternion to Rotation Matrix
      mask Display:
      | text(0.5, 0.5, '{\bfPRISMA}','horizontalAlignment','center','verticalAlignment','bottom','texmode','on');
      | text(0.5, 0.5, 'Quaternion to Rotation Matrix','horizontalAlignment','center','verticalAlignment','top');
  Transform Position NED to OpenGL : Subsystem
      mask help: Transform a three-dimensional position from the NED frame to the OpenGL frame.
      mask DialogControl DescGroupVar Prompt: Transform Position NED to OpenGL
      mask Display:
      | text(0.5, 0.5, '{\bfPosition}','horizontalAlignment','center','verticalAlignment','bottom','texmode','on');
      | text(0.5, 0.5, 'NED to OpenGL','horizontalAlignment','center','verticalAlignment','top');
  Transform Position OpenGL to NED : Subsystem
      mask help: Transform a three-dimensional position from the OpenGL frame to the NED frame.
      mask DialogControl DescGroupVar Prompt: Transform Position OpenGL to NED
      mask Display:
      | text(0.5, 0.5, '{\bfPosition}','horizontalAlignment','center','verticalAlignment','bottom','texmode','on');
      | text(0.5, 0.5, 'OpenGL to NED','horizontalAlignment','center','verticalAlignment','top');
  Transform Quaternion NED to OpenGL : Subsystem
      mask help: Transform a unit quaternion from the NED frame to the OpenGL frame. The unit quaternion is given by the components [w;x;y;z], where w denotes the scalar part and [x;y;z] indicates the vector part.
      mask DialogControl DescGroupVar Prompt: Transform Quaternion NED to OpenGL
      mask Display:
      | text(0.5, 0.5, '{\bfQuaternion}','horizontalAlignment','center','verticalAlignment','bottom','texmode','on');
      | text(0.5, 0.5, 'NED to OpenGL','horizontalAlignment','center','verticalAlignment','top');
  Transform Quaternion OpenGL to NED : Subsystem
      mask help: Transform a unit quaternion from the OpenGL frame to the NED frame. The unit quaternion is given by the components [w;x;y;z], where w denotes the scalar part and [x;y;z] indicates the vector part.
      mask DialogControl DescGroupVar Prompt: Transform Quaternion OpenGL to NED
      mask Display:
      | text(0.5, 0.5, '{\bfQuaternion}','horizontalAlignment','center','verticalAlignment','bottom','texmode','on');
      | text(0.5, 0.5, 'OpenGL to NED','horizontalAlignment','center','verticalAlignment','top');
  Transform Scale NED to OpenGL : Subsystem
      mask help: Transform a three-dimensional scale from the NED frame to the OpenGL frame.
      mask DialogControl DescGroupVar Prompt: Transform Scale NED to OpenGL
      mask Display:
      | text(0.5, 0.5, '{\bfScale}','horizontalAlignment','center','verticalAlignment','bottom','texmode','on');
      | text(0.5, 0.5, 'NED to OpenGL','horizontalAlignment','center','verticalAlignment','top');
  Transform Scale OpenGL to NED : Subsystem
      mask help: Transform a three-dimensional scale from the OpenGL frame to the NED frame.
      mask DialogControl DescGroupVar Prompt: Transform Scale OpenGL to NED
      mask Display:
      | text(0.5, 0.5, '{\bfScale}','horizontalAlignment','center','verticalAlignment','bottom','texmode','on');
      | text(0.5, 0.5, 'OpenGL to NED','horizontalAlignment','center','verticalAlignment','top');

== system PRISMA/Unpack Window Event Message ==
  bytes : Inport  OutDataTypeStr=uint8
  length : Inport  Port=2  OutDataTypeStr=int32  PortDimensions=1
  AND : Logic  AllPortsSameDT=off  OutDataTypeStr=boolean
  Compare To Constant : simulink/Logic and Bit Operations/Compare To Constant  relop=>=  const=int32(19)  OutDataTypeStr=boolean
  Min : MinMax  Inputs=2
  Width : Width  DataType=int32
  unpack : Subsystem  TreatAsAtomicUnit=on
  success : Outport  OutDataTypeStr=boolean  PortDimensions=1
  windowEvent : Outport  Port=2
  wires:
  bytes/1 -> unpack/2(bytes), Width/1
  Width/1 -> Min/2
  length/1 -> Min/1
  Min/1 -> unpack/1(length), Compare To Constant/1
  Compare To Constant/1 -> AND/1, unpack/Enable
  unpack/1(success) -> AND/2
  AND/1 -> success/1
  unpack/2(windowEvent) -> windowEvent/1

== system PRISMA/details ==
  PRISMA Bitfield To Byte : Subsystem
      mask help: Convert a bitfield of 8 boolean values to one byte.
      mask DialogControl DescGroupVar Prompt: PRISMA Bitfield To Byte
      mask Display:
      | text(0.5, 0.5, '{\bfPRISMA}','horizontalAlignment','center','verticalAlignment','bottom','texmode','on');
      | text(0.5, 0.5, 'Bitfield to Byte','horizontalAlignment','center','verticalAlignment','top');
  PRISMA Message Type : Subsystem  mask{messageType=Clear}
      mask prompts: messageType "Message Type:"
      mask help: Create the byte representing a specific message type.
      mask TypeOptions messageType: Clear | Engine Parameter | Camera | Atmosphere | Ambient Light | Directional Light | Point Light | Spot Light | Mesh | Watermesh | Dynamic Mesh
      mask DialogControl DescGroupVar Prompt: PRISMA Message Type
      mask Display:
      | maskStr = get_param(gcb,'messageType');
      | strText = ['Message Type: ' maskStr];
      | text(0.05, 0.5, '{\bfPRISMA}','horizontalAlignment','left','verticalAlignment','bottom','texmode','on');
      | text(0.05, 0.5, strText,'horizontalAlignment','left','verticalAlignment','top');
  Swap Double Native To Network : Subsystem
      mask help: Swap bytes of the input value from native byte-order to network byte-order or vice versa.
      mask DialogControl DescGroupVar Prompt: Swap Double Native To Network
      mask Display:
      | text(0.5, 0.5, '{\bfPRISMA}','horizontalAlignment','center','verticalAlignment','bottom','texmode','on');
      | text(0.5, 0.5, 'Swap Double Native To Network','horizontalAlignment','center','verticalAlignment','top');
  Swap Float Native To Network : Subsystem
      mask help: Swap bytes of the input value from native byte-order to network byte-order or vice versa.
      mask DialogControl DescGroupVar Prompt: Swap Float Native To Network
      mask Display:
      | text(0.5, 0.5, '{\bfPRISMA}','horizontalAlignment','center','verticalAlignment','bottom','texmode','on');
      | text(0.5, 0.5, 'Swap Float Native To Network','horizontalAlignment','center','verticalAlignment','top');
  Swap Int32 Native To Network : Subsystem
      mask help: Swap bytes of the input value from native byte-order to network byte-order or vice versa.
      mask DialogControl DescGroupVar Prompt: Swap Int32 Native To Network
      mask Display:
      | text(0.5, 0.5, '{\bfPRISMA}','horizontalAlignment','center','verticalAlignment','bottom','texmode','on');
      | text(0.5, 0.5, 'Swap Int32 Native To Network','horizontalAlignment','center','verticalAlignment','top');
  Swap Uint16 Native To Network : Subsystem
      mask help: Swap bytes of the input value from native byte-order to network byte-order or vice versa.
      mask DialogControl DescGroupVar Prompt: Swap Uint16 Native To Network
      mask Display:
      | text(0.5, 0.5, '{\bfPRISMA}','horizontalAlignment','center','verticalAlignment','bottom','texmode','on');
      | text(0.5, 0.5, 'Swap Uint16 Native To Network','horizontalAlignment','center','verticalAlignment','top');
  Swap Uint32 Native To Network : Subsystem
      mask help: Swap bytes of the input value from native byte-order to network byte-order or vice versa.
      mask DialogControl DescGroupVar Prompt: Swap Uint32 Native To Network
      mask Display:
      | text(0.5, 0.5, '{\bfPRISMA}','horizontalAlignment','center','verticalAlignment','bottom','texmode','on');
      | text(0.5, 0.5, 'Swap Uint32 Native To Network','horizontalAlignment','center','verticalAlignment','top');

== system PRISMA/Transformation/Euler ZYX to Quaternion ==
  roll : Inport  OutDataTypeStr=double  Unit=rad  PortDimensions=1
  pitch : Inport  Port=2  OutDataTypeStr=double  Unit=rad  PortDimensions=1
  yaw : Inport  Port=3  OutDataTypeStr=double  Unit=rad  PortDimensions=1
  MATLAB Function : MATLAB Function  TreatAsAtomicUnit=on
  q : Outport  OutDataTypeStr=double  PortDimensions=4
  wires:
  roll/1 -> MATLAB Function/1(roll)
  MATLAB Function/1(q) -> q/1
  pitch/1 -> MATLAB Function/2(pitch)
  yaw/1 -> MATLAB Function/3(yaw)

== system PRISMA/Transformation/Look At to Quaternion ==
  eyePosition : Inport  OutDataTypeStr=double  PortDimensions=3
  lookAtPosition : Inport  Port=2  OutDataTypeStr=double  PortDimensions=3
  MATLAB Function : MATLAB Function  TreatAsAtomicUnit=on
  quaternion : Outport  OutDataTypeStr=double  PortDimensions=4
  wires:
  eyePosition/1 -> MATLAB Function/1(eyePosition)
  lookAtPosition/1 -> MATLAB Function/2(lookAtPosition)
  MATLAB Function/1(quaternion) -> quaternion/1

== system PRISMA/Transformation/Quaternion to Rotation Matrix ==
  quaternion : Inport  OutDataTypeStr=double  PortDimensions=4
  MATLAB Function : MATLAB Function  TreatAsAtomicUnit=on
  rotationMatrix : Outport  OutDataTypeStr=double  PortDimensions=[3 3]
  wires:
  MATLAB Function/1(dcm) -> rotationMatrix/1
  quaternion/1 -> MATLAB Function/1(q)

== system PRISMA/Transformation/Transform Position NED to OpenGL ==
  NED : Inport  OutDataTypeStr=double  PortDimensions=3
  Mux : Mux  Inputs=3
  Selector : Selector  InputPortWidth=3  IndexOptions=Index vector (dialog)  Indices=2  OutputSizes=1
  Selector1 : Selector  InputPortWidth=3  IndexOptions=Index vector (dialog)  Indices=1  OutputSizes=1
  Selector2 : Selector  InputPortWidth=3  IndexOptions=Index vector (dialog)  Indices=3  OutputSizes=1
  Unary Minus : UnaryMinus
  Unary Minus1 : UnaryMinus
  OpenGL : Outport  OutDataTypeStr=double  PortDimensions=3
  wires:
  NED/1 -> Selector2/1, Selector1/1, Selector/1
  Mux/1 -> OpenGL/1
  Selector/1 -> Mux/1
  Unary Minus/1 -> Mux/2
  Selector1/1 -> Unary Minus1/1
  Selector2/1 -> Unary Minus/1
  Unary Minus1/1 -> Mux/3

== system PRISMA/Transformation/Transform Position OpenGL to NED ==
  OpenGL : Inport  OutDataTypeStr=double  PortDimensions=3
  Mux : Mux  Inputs=3
  Selector : Selector  InputPortWidth=3  IndexOptions=Index vector (dialog)  Indices=2  OutputSizes=1
  Selector1 : Selector  InputPortWidth=3  IndexOptions=Index vector (dialog)  Indices=1  OutputSizes=1
  Selector2 : Selector  InputPortWidth=3  IndexOptions=Index vector (dialog)  Indices=3  OutputSizes=1
  Unary Minus1 : UnaryMinus
  Unary Minus2 : UnaryMinus
  NED : Outport  OutDataTypeStr=double  PortDimensions=3
  wires:
  Selector1/1 -> Mux/2
  Unary Minus1/1 -> Mux/3
  Selector/1 -> Unary Minus1/1
  Selector2/1 -> Unary Minus2/1
  Mux/1 -> NED/1
  OpenGL/1 -> Selector2/1, Selector1/1, Selector/1
  Unary Minus2/1 -> Mux/1

== system PRISMA/Transformation/Transform Quaternion NED to OpenGL ==
  NED : Inport  OutDataTypeStr=double  PortDimensions=4
  Mux : Mux
  Selector : Selector  InputPortWidth=4  IndexOptions=Index vector (dialog)  Indices=3  OutputSizes=1
  Selector1 : Selector  InputPortWidth=4  IndexOptions=Index vector (dialog)  Indices=2  OutputSizes=1
  Selector2 : Selector  InputPortWidth=4  IndexOptions=Index vector (dialog)  Indices=4  OutputSizes=1
  Selector3 : Selector  InputPortWidth=4  IndexOptions=Index vector (dialog)  Indices=1  OutputSizes=1
  Unary Minus : UnaryMinus
  Unary Minus1 : UnaryMinus
  OpenGL : Outport  OutDataTypeStr=double  PortDimensions=4
  wires:
  Selector3/1 -> Mux/1
  Selector2/1 -> Unary Minus/1
  Selector1/1 -> Unary Minus1/1
  Unary Minus/1 -> Mux/3
  Selector/1 -> Mux/2
  Mux/1 -> OpenGL/1
  NED/1 -> Selector/1, Selector3/1, Selector1/1, Selector2/1
  Unary Minus1/1 -> Mux/4
